simulink model "A239"  (R2018b)
settings: Solver=FixedStepAuto  StartTime=0.0  StopTime=10.0  RelTol=1e-3  EnableMultiTasking=on
undefined symbols (not defined in the file): k1, k2, piConst, tau
libraries: arduinolib x1, simulink x1
settings Model: SimulationMode=external  ExtModeTrigDuration=2  Creator=bill  LastModifiedBy=bill
settings OptimizationCC: EnhancedBackFolding=on  PassReuseOutputArgsAs=Individual arguments  MaxStackSize=64  OptimizeBlockOrder=speed  DifferentSizesBufferReuse=on  OptimizationCustomize=off
settings DebuggingCC: ParameterTunabilityLossMsg=error
settings HardwareCC: ProdBitPerInt=16  ProdBitPerPointer=16  ProdBitPerSizeT=16  ProdBitPerPtrDiffT=16  ProdLargestAtomicFloat=None  ProdWordSize=8  ProdHWDeviceType=Atmel->AVR  UseEmbeddedCoderFeatures=off  UseSimulinkCoderFeatures=off
settings SFSimCC: MATLABDynamicMemAlloc=off
settings RTWCC: SystemTargetFile=ert.tlc  HardwareBoard=Arduino Uno  TemplateMakefile=ert_default_tmf  GenerateReport=on  Toolchain=Arduino AVR  BuildConfiguration=Faster Runs  IncludeHyperlinkInReport=on  LaunchReport=on  GenerateTraceInfo=on  GenerateTraceReport=on  GenerateTraceReportSl=on  GenerateTraceReportSf=on  GenerateTraceReportEml=on
settings CodeAppCC: ForceParamTrailComments=on  IgnoreCustomStorageClasses=off  OperatorAnnotations=on  SimulinkDataObjDesc=on  SFDataObjDesc=on  InsertBlockDesc=on
settings ERTTargetCC: SupportContinuousTime=on  SupportNonInlinedSFcns=on  SupportVariableSizeSignals=on

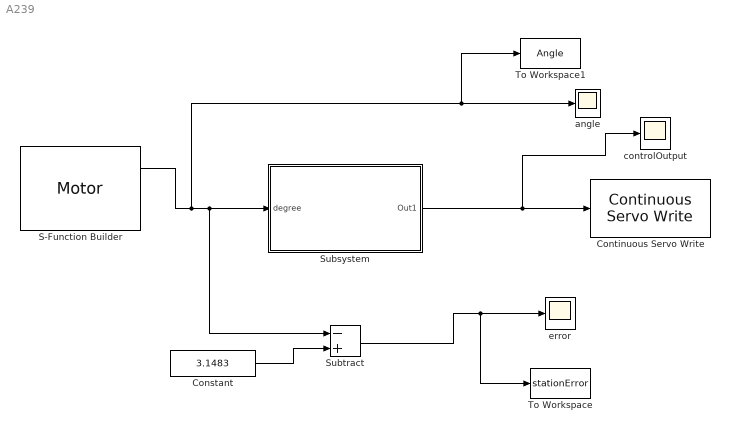
== system A239 ==
  Constant : Constant  Value=3.1483
  Continuous Servo Write : arduinolib/Continuous Servo Write  pinNumber=7  ServoIndex=0  blockPlatform=ARDUINO
      settings: SourceProductName=Simulink Support Package for Arduino Hardware  SourceProductBaseCode=ARDUINO
  S-Function Builder : S-Function  InitFcn=try, set_param(gcb,'FunctionName','Motor'), end  FunctionName=Motor  SFunctionModules=Motor_wrapper  SFunctionDeploymentMode=off  EnableBusSupport=off  mask(S-Function Builder){}
      mask help: Simulink:masks:SFunctionBuilder_MD
      mask init:
      | val = [[.9  0.75 0.75 1 1 .9 .9 1]',[1 1 0.75 0.75 .9 .9 1 .9]'];try , sys = get_param(gcb,'SfunBuilderFcnName');if isempty(sys), sys = get_param(gcb,'FunctionName'); end,catch, sys = get_param(gcb,'FunctionName'); end
      settings: CopyFcn=set_param(gcbh,'LinkStatus','none')  PreSaveFcn=try, set_param(gcb,'FunctionName','Motor'), end  OpenFcn=sfunctionwizard(gcbh)
      mask Display: plot(val(:,1),val(:,2)),disp(sys), port_label('output',1,'posRad'), port_label('output',2,'deriv')
  Subsystem : Subsystem
  Subtract : Sum  Inputs=-+
  To Workspace : ToWorkspace  VariableName=stationError  SampleTime=-1
  To Workspace1 : ToWorkspace  VariableName=Angle  SampleTime=-1
  angle : Scope
  controlOutput : Scope
  error : Scope
  wires:
  Subsystem/1(Out1) -> controlOutput/1, Continuous Servo Write/1
  S-Function Builder/1 -> To Workspace1/1, angle/1, Subtract/1, Subsystem/1(degree)
  Constant/1 -> Subtract/2
  Subtract/1 -> To Workspace/1, error/1

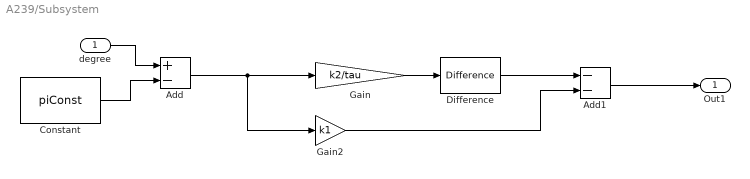
== system A239/Subsystem ==
  degree : Inport
  Add : Sum  Inputs=+-
  Add1 : Sum  Inputs=--
  Constant : Constant  Value=piConst
  Difference : simulink/Discrete/Difference  ICPrevInput=0.0  OutMin=[]  OutMax=[]  OutDataType=fixdt(1, 16)  OutScaling=2^-10  DoSatur=off
  Gain : Gain  Gain=k2/tau
  Gain2 : Gain  Gain=k1
  Out1 : Outport
  wires:
  degree/1 -> Add/1
  Add1/1 -> Out1/1
  Difference/1 -> Add1/1
  Constant/1 -> Add/2
  Gain/1 -> Difference/1
  Add/1 -> Gain/1, Gain2/1
  Gain2/1 -> Add1/2
